simulink model "SM_simulation"  (R2022b)
settings: Solver=VariableStepAuto  StartTime=0.0  StopTime=30  MaxStep=1e-4  RelTol=1e-3
values from neighbouring files (symbols this model uses):
  Kd_zn = (Kp_zn*T)/8    (= 0.33)    [tuning.m]
  Ki_zn = (2*Kp_zn)/T    (= 0.272727272727)    [tuning.m]
  Kp_zn = 0.6*Ku    (= 0.6)    [tuning.m]
undefined symbols (not defined in the file or in its folder): DiscIntNeverNeededParam, Kd, Ki
libraries: simulink x4, slpidlib x1
settings Model: Creator=NYINYI  LastModifiedBy=nyinyia
settings SolverCC: ZeroCrossAlgorithm=Adaptive
settings DebuggingCC: IgnoredZcDiagnostic=none

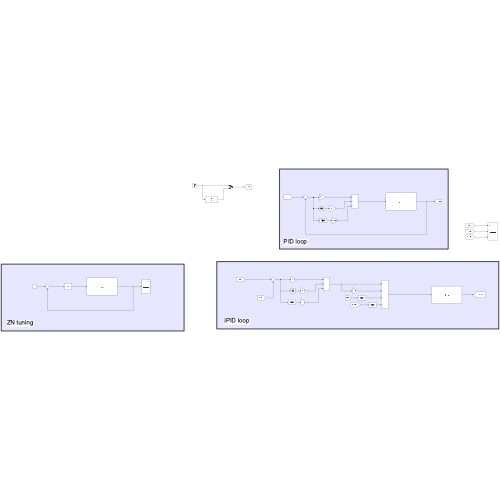
[thumbnail: Simulink's stored preview of the top-level diagram]
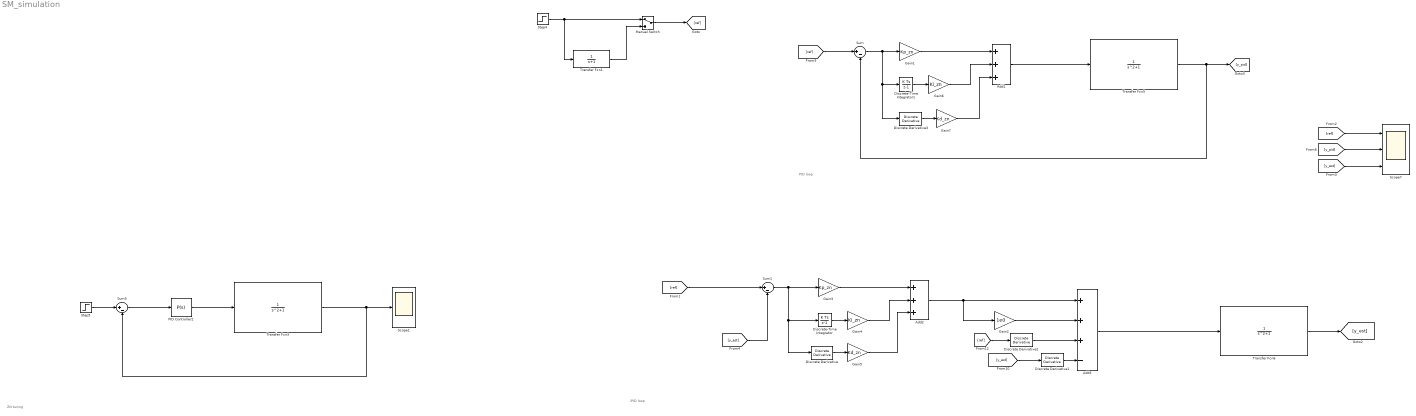
== system SM_simulation ==
  note: iPID loop
  note: ZN tuning
  note: PID loop
  Add1 : Sum  Inputs=+++
  Add2 : Sum  Inputs=+++
  Add3 : Sum  Inputs=+++-
  Discrete Derivative{,1..3} (4 alike) : simulink/Discrete/Discrete Derivative  gainval=1.0  ICPrevScaledInput=0.0  OutMin=[]  OutMax=[]  OutDataType=fixdt(1, 16)  OutScaling=2^-10  DoSatur=off
  Discrete-Time Integrator : DiscreteIntegrator  SampleTime=-1  ICPrevOutput=DiscIntNeverNeededParam  ICPrevScaledInput=DiscIntNeverNeededParam
  Discrete-Time Integrator1 : DiscreteIntegrator  SampleTime=-1  ICPrevOutput=DiscIntNeverNeededParam  ICPrevScaledInput=DiscIntNeverNeededParam
  Gain1 : Gain  Gain=Kp_zn
  Gain2 : Gain  Gain=1e0
  Gain3 : Gain  Gain=Kp_zn
  Gain4 : Gain  Gain=Ki_zn
  Gain5 : Gain  Gain=Kd_zn
  Gain6 : Gain  Gain=Ki_zn
  Gain7 : Gain  Gain=Kd_zn
  Manual Switch : ManualSwitch
  PID Controller2 : slpidlib/PID Controller  Controller=P  Form=Parallel  TimeDomain=Continuous-time  UseExternalTs=off  SampleTime=-1  IntegratorMethod=Forward Euler  FilterMethod=Forward Euler  ControllerParametersSource=internal  P=1  I=Ki  UseKiTs=off  D=Kd  N=31.0667370516641  UseFilter=on  TunerSelectOption=Transfer Function Based (PID Tuner App)  InitialConditionSource=internal  InitialConditionForIntegrator=0  InitialConditionForFilter=0  DifferentiatorICPrevScaledInput=0  ExternalReset=none  TrackingMode=off  Kt=1  LimitOutput=off  SatLimitsSource=internal  UpperSaturationLimit=inf  LowerSaturationLimit=-inf  LinearizeAsGain=on  AntiWindupMode=none  Kb=1  LimitIntegrator=off  UpperIntegratorSaturationLimit=inf  LowerIntegratorSaturationLimit=-inf  POutMin=[]  POutMax=[]  IOutMin=[]  IOutMax=[]  DOutMin=[]  DOutMax=[]  NOutMin=[]  NOutMax=[]  SumOutMin=[]  SumOutMax=[]  SaturationOutMin=[]  SaturationOutMax=[]  PParamMin=[]  PParamMax=[]  IParamMin=[]  IParamMax=[]  DParamMin=[]  DParamMax=[]  NParamMin=[]  NParamMax=[]  KbParamMin=[]  KbParamMax=[]  KtParamMin=[]  KtParamMax=[]  KbOutMin=[]  KbOutMax=[]  KtOutMin=[]  KtOutMax=[]  IntegratorOutMin=[]  IntegratorOutMax=[]  FilterOutMin=[]  FilterOutMax=[]  SumI1OutMin=[]  SumI1OutMax=[]  SumI2OutMin=[]  SumI2OutMax=[]  SumI3OutMin=[]  SumI3OutMax=[]  SumI4OutMin=[]  SumI4OutMax=[]  SumDOutMin=[]  SumDOutMax=[]  DifferentiatorOutMin=[]  DifferentiatorOutMax=[]  FilterDiffOutCoefMin=[]  FilterDiffOutCoefMax=[]  ReciprocalOutMin=[]  ReciprocalOutMax=[]  SumDenOutMin=[]  SumDenOutMax=[]  SumNumOutMin=[]  SumNumOutMax=[]  DivideOutMin=[]  DivideOutMax=[]  UdiffTsProdOutMin=[]  UdiffTsProdOutMax=[]  NTsProdOutMin=[]  NTsProdOutMax=[]  UintegralTsProdOutMin=[]  UintegralTsProdOutMax=[]  UngainTsProdOutMin=[]  UngainTsProdOutMax=[]  ClampingZeroOutDataTypeStr=Inherit: Inherit via back propagation  ClampingZeroOutMin=[]  ClampingZeroOutMax=[]  FilterDenConstantOutDataTypeStr=Inherit: Inherit via back propagation  FilterDenConstantOutMin=[]  FilterDenConstantOutMax=[]  PCopyOutDataTypeStr=Inherit: Inherit via back propagation  PCopyOutMin=[]  PCopyOutMax=[]  NCopyOutDataTypeStr=Inherit: Inherit via back propagation  NCopyOutMin=[]  NCopyOutMax=[]  IntegratorContinuousStateAttributes=''  IntegratorStateMustResolveToSignalObject=off  IntegratorRTWStateStorageClass=Auto  FilterContinuousStateAttributes=''  FilterStateMustResolveToSignalObject=off  FilterRTWStateStorageClass=Auto  ParallelPVariant=InternalParameters  IdealPVariant=Disabled  IVariant=Disabled  DVariant=Disabled  IntegratorVariant=Disabled  SatVariant=Disabled  AWVariant=Disabled  PCopyVariant=Disabled  TRVariant=Disabled  FdbkBlocksVariant=Forward  IdealPFdbkVariant=Disabled  SatFdbkVariant=Disabled  DerivativeFilterVariant=Disabled  NVariant=Disabled  NCopyVariant=Disabled_SignalSpec  FilterICVariant=Disabled  IntegratorICVariant=Disabled  ExternalResetVariant=Disabled  TRSumVariant=Passthrough  SumFdbkVariant=Disabled  SumVariant=Passthrough_P  TsampFilterVariant=InternalTs  TsampNgainVariant=Passthrough  TsampIntegralVariant=Disabled_SignalSpec  ExternalSaturationOutDataTypeStr=Inherit: Same as second input
  Scope1 : Scope
  Scope7 : Scope  NumInputPorts=3
  Step4 : Step  SampleTime=0
  Step5 : Step  SampleTime=0
  Sum : Sum  Inputs=|+-
  Sum1 : Sum  Inputs=|+-
  Sum5 : Sum  Inputs=|+-
  Transfer Fcn1 : TransferFcn  Denominator=[1 1]
  Transfer Fcn3 : TransferFcn  Denominator=[1 0 1]
  Transfer Fcn5 : TransferFcn  Denominator=[1 0 1]
  Transfer Fcn6 : TransferFcn  Denominator=[1 0 1]
  wires:
  Transfer Fcn5/1 -> Sum/2, [y_pid]
  Sum/1 -> Discrete Derivative3/1, Discrete-Time Integrator1/1, Gain1/1
  [ref] -> Sum1/1
  Transfer Fcn6/1 -> [y_est]
  [ref] -> Sum/1
  Manual Switch/1 -> [ref]
  Step4/1 -> Transfer Fcn1/1, Manual Switch/1
  Transfer Fcn1/1 -> Manual Switch/2
  PID Controller2/1 -> Transfer Fcn3/1
  Transfer Fcn3/1 -> Scope1/1, Sum5/2
  Step5/1 -> Sum5/1
  Sum5/1 -> PID Controller2/1
  Gain2/1 -> Add3/2
  [y_est] -> Discrete Derivative1/1
  [ref] -> Discrete Derivative2/1
  Discrete Derivative2/1 -> Add3/3
  Discrete Derivative1/1 -> Add3/4
  Add3/1 -> Transfer Fcn6/1
  Discrete Derivative/1 -> Gain5/1
  Discrete-Time Integrator/1 -> Gain4/1
  Sum1/1 -> Discrete-Time Integrator/1, Discrete Derivative/1, Gain3/1
  Gain3/1 -> Add2/1
  Gain4/1 -> Add2/2
  Gain5/1 -> Add2/3
  Add2/1 -> Gain2/1, Add3/1
  Add1/1 -> Transfer Fcn5/1
  Gain7/1 -> Add1/3
  Gain6/1 -> Add1/2
  Gain1/1 -> Add1/1
  Discrete-Time Integrator1/1 -> Gain6/1
  Discrete Derivative3/1 -> Gain7/1
  [y_est] -> Scope7/3
  [y_est] -> Sum1/2
  [y_pid] -> Scope7/2
  [ref] -> Scope7/1
